simulink model "GasTurbine_SS_Template"  (R2019b)
settings: Solver=FixedStepDiscrete  StartTime=0.0  StopTime=MWS.in.SimTime  FixedStep=MWS.Solve.T  RelTol=1e-3  EnableMultiTasking=on
undefined symbols (not defined in the file): stripchar_TMATS
libraries: Lib_Turbo_Ambient_TMATS x1, Lib_Turbo_Burner_TMATS x1, Lib_Turbo_Compressor_TMATS x1, Lib_Turbo_Duct_TMATS x1, Lib_Turbo_Inlet_TMATS x1, Lib_Turbo_Nozzle_TMATS x1, Lib_Solve_SSNRSolverJC_TMATS x1, Lib_Turbo_Shaft_TMATS x1, Lib_Turbo_Turbine_TMATS x1
CloseFcn:
  | run(strcat(MWS.top_level, filesep,'GasTurbine_SS_Example_cleanup'))
settings Model: Creator=jwchapm2  LastModifiedBy=bhisma
settings DataIOCC: LimitDataPoints=on  SaveFormat=Array  SaveOutput=off  SaveTime=off  ReturnWorkspaceOutputs=off  SignalLoggingName=SimulationOutput
settings OptimizationCC: BlockReduction=off  DefaultParameterBehavior=Inlined  BufferReuse=off  ExpressionDepthLimit=2147483647  LifeSpan=inf
settings DebuggingCC: UnderspecifiedInitializationDetection=Classic  MergeDetectMultiDrivingBlocksExec=none  SolverPrmCheckMsg=warning  StateNameClashWarn=warning  SFUnexpectedBacktrackingDiag=warning  SFNoUnconditionalDefaultTransitionDiag=warning  SFExecutionAtInitializationDiag=none  ArithmeticOperatorsInVariantConditions=warning
settings HardwareCC: ProdBitPerPointer=32  ProdBitPerSizeT=32  ProdBitPerPtrDiffT=32  ProdLargestAtomicFloat=None  ProdIntDivRoundTo=Undefined  ProdEndianess=Unspecified  ProdWordSize=32  ProdHWDeviceType=32-bit Generic
settings ModelReferenceCC: PropagateSignalLabelsOutOfModel=off
settings SFSimCC: SimUseLocalCustomCode=off  CustomCodeUndefinedFunction=UseInterfaceOnly
settings RTWCC: RTWUseLocalCustomCode=off
settings CodeAppCC: StateflowObjectComments=on
settings GRTTargetCC: TargetLangStandard=C89/C90 (ANSI)  GeneratePreprocessorConditionals=Disable all
settings ConfigComp: CovMetricSettings=dw  CovHtmlReporting=on  CovSaveCumulativeToWorkspaceVar=on  CovSaveSingleToWorkspaceVar=on  CovExternalEMLEnable=off

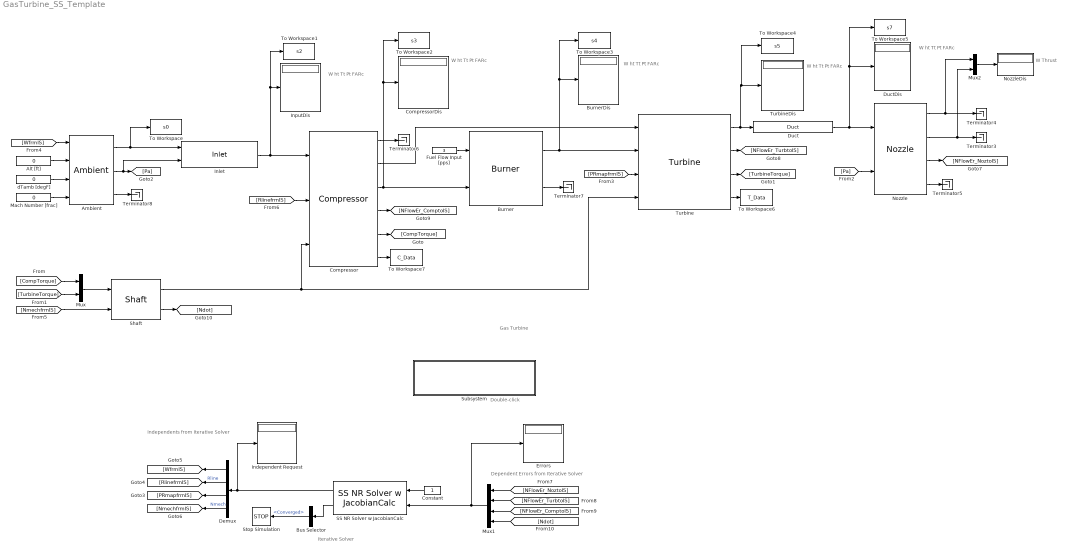
== system GasTurbine_SS_Template ==
  note: Double-click
  note: Independents from Iterative Solver
  note: W
      | ht
      | Tt
      | Pt
      | FARc
  note: W
      | Thrust
  note: W
      | ht
      | Tt
      | Pt
      | FARc
  note: W
      | ht
      | Tt
      | Pt
      | FARc
  note: W
      | ht
      | Tt
      | Pt
      | FARc
  note: W
      | ht
      | Tt
      | Pt
      | FARc
  note: Dependent Errors from Iterative Solver
  note: Iterative Solver
  note: Gas Turbine
  Alt [ft] : Constant  Value=0
  Ambient : Lib_Turbo_Ambient_TMATS/Ambient  X_A_AltVec_M=5000*[-1 0 1 2 3 4 5 6 7 8 9 10 12 14 16]  T_A_TsVec_M=[536.51 518.67 500.84 483.03 465.22 447.41 429.62 411.84 394.06 389.97 389.97 389.97 389.97 392.25 397.69]  T_A_PsVec_M=[17.554 14.696 12.228 10.108 8.297 6.759 5.461 4.373 3.468 2.73 2.149 1.692 1.049 0.651 0.406]  AFARc_M=0  X_A_FARVec_M=[0; 0.0050; 0.0100; 0.0150; 0.0200; 0.0250; 0.0300]  T_A_RtArray_M="[0.0686;    0.0686;    0.0686;    0.0686;    0.0686;    0.0686;    0.0686]"  Y_A_TVec_M=[300 10000]  T_A_gammaArray_M=[ 1.4 1.4 1.4 1.4 1.4 1.4 1.4; 1.4 1.4 1.4 1.4 1.4 1.4 1.4]
  Burner : Lib_Turbo_Burner_TMATS/Burner  LHVEn_M=on  LHV_M=MWS.Burner.LHV  Eff_M=1  hFuel_M=-1200  dPnormBurner_M=MWS.Burner.dP
  BurnerDis : Display
  Bus Selector : BusSelector  OutputSignals=Converged
  Compressor : Lib_Turbo_Compressor_TMATS/Compressor  X_C_RlineVec_M=MWS.HPC.RlineVec  Z_C_AlphaVec_M=1  Y_C_Map_NcVec_M=MWS.HPC.NcVec  T_C_Map_WcArray_M=MWS.HPC.WcArray  T_C_Map_PRArray_M=MWS.HPC.PRArray  T_C_Map_EffArray_M=MWS.HPC.EffArray  s_C_Nc_M=MWS.HPC.s_Nc  s_C_Wc_M=MWS.HPC.s_Wc  s_C_PR_M=MWS.HPC.s_PR  s_C_Eff_M=MWS.HPC.s_eff  SL_M=off  Scale_M=none  CBLDEN_M=off  C_CBD_M=0  C_CBFht_M=0.5  C_CBFPt_M=0.5  FBLDEN_M=off  C_FBD_M=0  C_BFht_M=0.5  C_BFPt_M=0.5  DefSMEn_M=off  SRline_M=1  X_C_Map_WcSurgeVec_M=MWS.HPC.WcMapSurge  T_C_Map_PRSurgeVec_M=MWS.HPC.PRMapSurge  iDesign_M=2  NcDes_M=1  EffDes_M=0.85  PRDes_M=20  RlineDes_M=2  FVar_M=strcat('iDes_',stripchar_TMATS(gcb),'.bin')  BlkNm_M=double(gcb)  HP_M=off
  CompressorDis : Display
  Constant : Constant
  Demux : Demux
  Duct : Lib_Turbo_Duct_TMATS/Duct  dP_M=MWS.Duct.dP
  DuctDis : Display
  Errors : Display
  Fuel Flow Input [pps] : Constant  Value=3
  Independent Request : Display
  Inlet : Lib_Turbo_Inlet_TMATS/Inlet  eRambase_M=MWS.Inlet.eRambase  X_eRamVec_M=[0 3]  T_eRamtbl_M=[1 1]
  InputDis : Display
  Mach Number [frac] : Constant  Value=0
  Mux : Mux  Inputs=2
  Mux1 : Mux
  Mux2 : Mux  Inputs=2
  Nozzle : Lib_Turbo_Nozzle_TMATS/Nozzle  SWType_M=Convergent  N_TArea_M=MWS.Noz.ATh  N_EArea_M=110.7  N_FL_M=MWS.Noz.LossPerc  X_N_TtVec2_M=MWS.Noz.TtVec  T_N_TGArray_M=MWS.Noz.TGArray  X_N_PEQPaVec_M=MWS.Noz.PeQPaVec  T_N_CdThArray_M=MWS.Noz.CdThArray  T_N_CvArray_M=MWS.Noz.CvArray  CfgEn_M=off  T_N_CfgArray_M=[1 1]  X_N_FARVec_M=MWS.Noz.FARVec  T_N_RtArray_M=MWS.Noz.RArray  Y_N_TtVec_M=MWS.Noz.TtVec  T_N_MAP_gammaArray_M=MWS.Noz.GArray  iDesign_M=2  WDes_M=103  FVar_M=strcat('iDes_',stripchar_TMATS(gcb),'.bin')
  NozzleDis : Display
  SS NR Solver w JacobianCalc : Lib_Solve_SSNRSolverJC_TMATS/SS NR Solver w JacobianCalc  SJac_Per_M=MWS.Solve.J_Calc_Per  SNR_IC_M=MWS.Solve.NR_IC  SNR_DX_M=MWS.Solve.NR_dx  SNR_Mx_M=100000  SNR_Mn_M=0.00001  SJacobianAttempts_M=MWS.Solve.NR_Jac_Re  Cond_Limits_M=MWS.Solve.C_Lim
  Shaft : Lib_Turbo_Shaft_TMATS/Shaft  Shaft_Inertia_M=MWS.Shaft.N_I
  Stop Simulation : Stop
  Subsystem : Subsystem
      settings: OpenFcn=run('PlotSSData.m')
      mask Display: fprintf('Plot Outputs')
  Terminator{3..8} (6 alike) : Terminator
  To Workspace : ToWorkspace  VariableName=s0  SaveFormat=Timeseries  SampleTime=-1
  To Workspace1 : ToWorkspace  VariableName=s2  SaveFormat=Timeseries  SampleTime=-1
  To Workspace2 : ToWorkspace  VariableName=s3  SaveFormat=Timeseries  SampleTime=-1
  To Workspace3 : ToWorkspace  VariableName=s4  SaveFormat=Timeseries  SampleTime=-1
  To Workspace4 : ToWorkspace  VariableName=s5  SaveFormat=Timeseries  SampleTime=-1
  To Workspace5 : ToWorkspace  VariableName=s7  SaveFormat=Timeseries  SampleTime=-1
  To Workspace6 : ToWorkspace  VariableName=T_Data  SaveFormat=Timeseries  SampleTime=-1
  To Workspace7 : ToWorkspace  VariableName=C_Data  SaveFormat=Timeseries  SampleTime=-1
  Turbine : Lib_Turbo_Turbine_TMATS/Turbine  X_T_Map_PRVec_M=MWS.HPT.PRVec  Y_T_Map_NcVec_M=MWS.HPT.NcVec  T_T_Map_WcArray_M=MWS.HPT.WcArray  T_T_Map_EffArray_M=MWS.HPT.EffArray  s_T_Nc_M=MWS.HPT.s_Nc  s_T_Wc_M=MWS.HPT.s_Wc  s_T_PR_M=MWS.HPT.s_PR  s_T_Eff_M=MWS.HPT.s_eff  ConfigNPSS_M=0  Scale_M=none  CFlwEn_M=off  T_CoolFlwPos_M=0  iDesign_M=2  NcDes_M=90  EffDes_M=0.9200  PRDes_M=5  NDes_M=10000  FVar_M=strcat('iDes_',stripchar_TMATS(gcb),'.bin')  BlkNm_M=double(gcb)  HP_M=off
  TurbineDis : Display
  dTamb [degF] : Constant  Value=0
  wires:
  Compressor/3 -> Burner/2, To Workspace2/1, CompressorDis/1
  Burner/2 -> Terminator7/1
  Nozzle/2 -> Terminator3/1, Mux2/2
  [Pa] -> Nozzle/2
  Burner/1 -> To Workspace3/1, BurnerDis/1, Turbine/2
  Turbine/1 -> To Workspace4/1, TurbineDis/1, Duct/1
  [PRmapfrmIS] -> Turbine/3
  Compressor/6 -> To Workspace7/1
  Turbine/4 -> To Workspace6/1
  Nozzle/1 -> Terminator4/1, Mux2/1
  Nozzle/4 -> Terminator5/1
  Inlet/1 -> To Workspace1/1, InputDis/1, Compressor/1
  Mux/1 -> Shaft/1
  Compressor/5 -> [CompTorque]
  Turbine/3 -> [TurbineTorque]
  [CompTorque] -> Mux/1
  [TurbineTorque] -> Mux/2
  Shaft/1 -> Compressor/3, Turbine/4
  Fuel Flow Input [pps]/1 -> Burner/1
  Mux1/1 -> SS NR Solver w JacobianCalc/2, Errors/1
  Demux/3 -> [PRmapfrmIS]
  Mux2/1 -> NozzleDis/1
  Duct/1 -> Nozzle/1, To Workspace5/1, DuctDis/1
  Compressor/1 -> Terminator6/1
  SS NR Solver w JacobianCalc/1 -> Independent Request/1, Demux/1
  Alt [ft]/1 -> Ambient/2
  Mach Number [frac]/1 -> Ambient/4
  Demux/1 -> [WfrmIS]
  Demux/2 -> [RlinefrmIS]  "Rline"
  Demux/4 -> [NmechfrmIS]  "Nmech"
  [WfrmIS] -> Ambient/1
  [NmechfrmIS] -> Shaft/2
  [RlinefrmIS] -> Compressor/2
  Nozzle/3 -> [NFlowEr_NoztoIS]
  [NFlowEr_NoztoIS] -> Mux1/1
  Turbine/2 -> [NFlowEr_TurbtoIS]
  [NFlowEr_TurbtoIS] -> Mux1/2
  Compressor/4 -> [NFlowEr_ComptoIS]
  [NFlowEr_ComptoIS] -> Mux1/3
  Shaft/2 -> [Ndot]
  [Ndot] -> Mux1/4
  Compressor/2 -> Turbine/1
  Ambient/2 -> Inlet/2, [Pa]
  Ambient/3 -> Terminator8/1
  dTamb [degF]/1 -> Ambient/3
  SS NR Solver w JacobianCalc/2 -> Bus Selector/1
  Constant/1 -> SS NR Solver w JacobianCalc/1
  Ambient/1 -> To Workspace/1, Inlet/1
  Bus Selector/1 -> Stop Simulation/1  "<Converged>"

== system GasTurbine_SS_Template/Subsystem ==
